simulink model "HW_FL"  (R2020b)
settings: Solver=FixedStepAuto  StartTime=0.0  StopTime=2  FixedStep=0.0001  RelTol=1e-3
undefined symbols (not defined in the file): a_filt, a_sin, b_filt, KdFL, KpFL, omega_sin, q_0_FL, q_dot_0_FL
settings Model: Creator=Alberto  LastModifiedBy=Musta

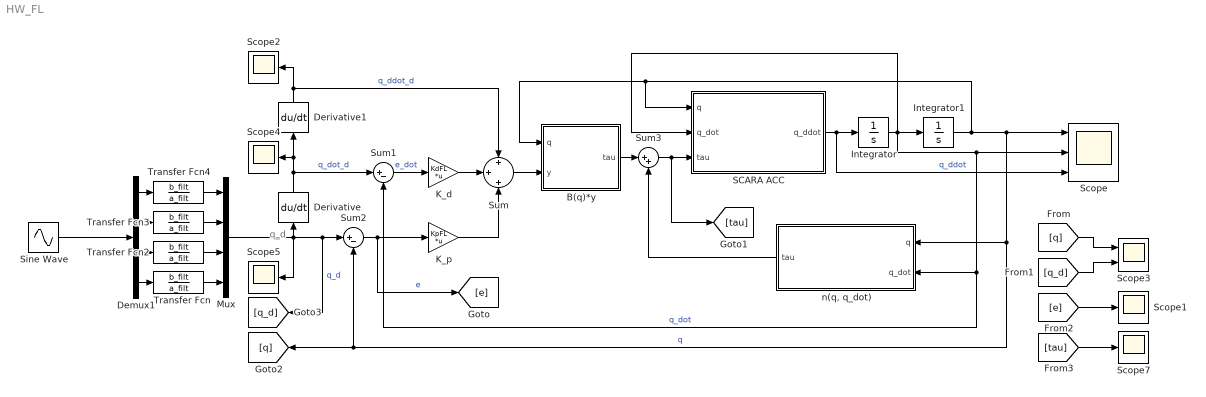
== system HW_FL ==
  note: q_d
  B(q)*y : MATLAB Function  TreatAsAtomicUnit=on
  Demux1 : Demux
  Derivative : Derivative
  Derivative1 : Derivative
  Integrator : Integrator  InitialCondition=q_dot_0_FL
  Integrator1 : Integrator  InitialCondition=q_0_FL
  K_d : Gain  Gain=KdFL  Multiplication=Matrix(K*u)
  K_p : Gain  Gain=KpFL  Multiplication=Matrix(K*u)
  Mux : Mux
  SCARA ACC : MATLAB Function  TreatAsAtomicUnit=on
  Scope : Scope  NumInputPorts=3
  Scope{1..2,4..5,7} (5 alike) : Scope
  Scope3 : Scope  NumInputPorts=2
  Sine Wave : Sin  Amplitude=a_sin  Frequency=omega_sin  SampleTime=0
  Sum : Sum  Inputs=+|+|+
  Sum1 : Sum  Inputs=|+-
  Sum2 : Sum  Inputs=|+-
  Sum3 : Sum  Inputs=|++
  Transfer Fcn{,2..4} (4 alike) : TransferFcn  Numerator=b_filt  Denominator=a_filt
  "n(q, q_dot)" : MATLAB Function  TreatAsAtomicUnit=on
  wires:
  SCARA ACC/1(q_ddot) -> Integrator/1, Scope/3  "q_ddot"
  Integrator/1 -> Integrator1/1, Scope/2, "n(q, q_dot)"/2(q_dot), Sum1/2, SCARA ACC/2(q_dot)  "q_dot"
  Integrator1/1 -> Scope/1, Sum2/2, [q], "n(q, q_dot)"/1(q), SCARA ACC/1(q), B(q)*y/1(q)  "q"
  Demux1/1 -> Transfer Fcn4/1
  Demux1/2 -> Transfer Fcn3/1
  Demux1/3 -> Transfer Fcn2/1
  Demux1/4 -> Transfer Fcn/1
  Transfer Fcn4/1 -> Mux/1
  Transfer Fcn3/1 -> Mux/2
  Transfer Fcn2/1 -> Mux/3
  Transfer Fcn/1 -> Mux/4
  Mux/1 -> Scope5/1, Derivative/1, [q_d], Sum2/1  "q_d"
  Sine Wave/1 -> Demux1/1
  Derivative/1 -> Derivative1/1, Scope4/1, Sum1/1  "q_dot_d"
  Derivative1/1 -> Sum/1, Scope2/1  "q_ddot_d"
  Sum1/1 -> K_d/1  "e_dot"
  Sum2/1 -> [e], K_p/1  "e"
  Sum3/1 -> [tau], SCARA ACC/3(tau)
  "n(q, q_dot)"/1(tau) -> Sum3/2
  B(q)*y/1(tau) -> Sum3/1
  Sum/1 -> B(q)*y/2(y)
  K_d/1 -> Sum/2
  K_p/1 -> Sum/3
  [q] -> Scope3/1
  [tau] -> Scope7/1
  [e] -> Scope1/1
  [q_d] -> Scope3/2

== matlab function HW_FL/SCARA ACC ==
  data: q input; q_ddot output; q_dot input; tau input
function q_ddot = SCARA_acc(q, q_dot, tau)%#codegen
    coder.extrinsic('f_B_mex'); 
    coder.extrinsic('f_C_vect_mex'); 
    coder.extrinsic('f_g_vect_mex');
    B = eye(4);
    C_vect = zeros(4,1);
    F_g = zeros(4,1);
    tau = reshape(tau,4,1);
    q_ddot = zeros(4,1);
    B = full(f_B_mex('f_B',q));
    C_vect = full(f_C_vect_mex('f_C_vect', q, q_dot));
    F_g = full(f_g_vect_mex('f_g_vect', q));
    q_ddot = (eye(4)/B)*(-C_vect-F_g+tau);
end

== matlab function HW_FL/n(q, q_dot) ==
  data: q input; tau output; q_dot input
function tau = n(q, q_dot)%#codegen
    coder.extrinsic('f_C_vect_mex'); 
    coder.extrinsic('f_g_vect_mex');
    C_vect = zeros(4,1);
    F_g = zeros(4,1);
    tau = zeros(4,1);
    C_vect = full(f_C_vect_mex('f_C_vect', q, q_dot));
    F_g = full(f_g_vect_mex('f_g_vect', q));
    tau = C_vect+F_g;
end

== matlab function HW_FL/B(q)*y ==
  data: q input; tau output; y input
function tau = B(q, y)%#codegen
    coder.extrinsic('f_B_mex'); 
    B = eye(4);
    tau = zeros(4,1);
    y = reshape(y,4,1);
    B = full(f_B_mex('f_B',q));
    tau = B*y;
end
